simulink model "LQR_fun"  (R2018a)
settings: Solver=ode1  StartTime=0.0  StopTime=30  FixedStep=0.001  RelTol=1e-3
InitFcn:
  | lqr_main
values from neighbouring files (symbols this model uses):
  den = [1 PlantX.B/PlantX.J PlantX.K/PlantX.J]    [lqr_m.m]    (also in lqr_main.m = [1 B/J K/J])
  num = [PlantX.K/PlantX.J]    [lqr_m.m]    (also in lqr_main.m = 15548.978804)
  tra_01 = tra_01'    [tra.m]
undefined symbols (not defined in the file or in its folder): DiscIntNeverNeededParam
libraries: simulink x3
settings Model: Creator=yuxi  LastModifiedBy=yuxi

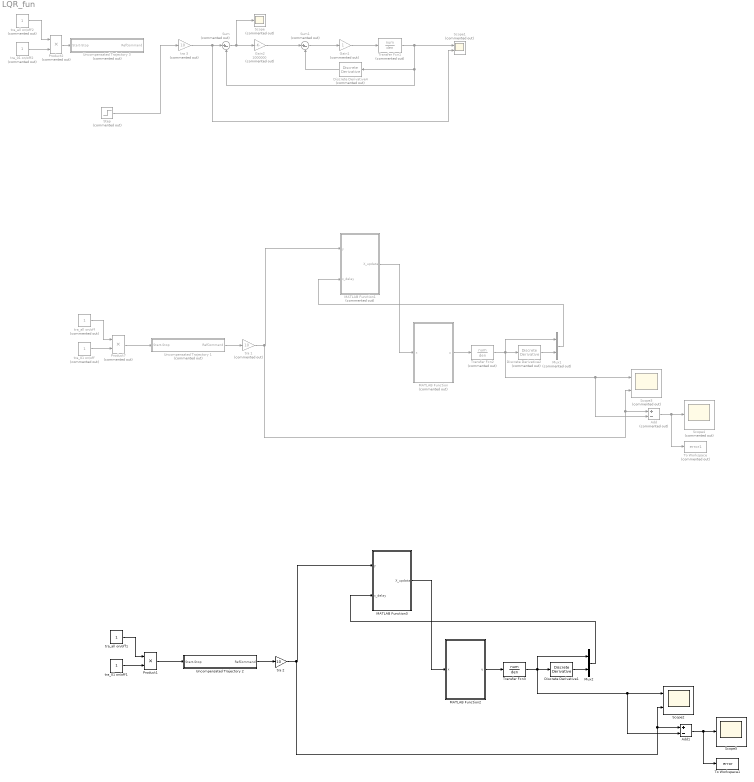
== system LQR_fun ==
  Add : Sum  Commented=on  Inputs=+-
  Add1 : Sum  Inputs=+-
  Discrete Derivative1 : simulink/Discrete/Discrete Derivative  gainval=1.0  ICPrevScaledInput=0.0  InputProcessing=Inherited  OutMin=[]  OutMax=[]  OutDataType=fixdt(1, 16)  OutScaling=2^-10  DoSatur=off
  Discrete Derivative2 : simulink/Discrete/Discrete Derivative  Commented=on  gainval=1.0  ICPrevScaledInput=0.0  InputProcessing=Inherited  OutMin=[]  OutMax=[]  OutDataType=fixdt(1, 16)  OutScaling=2^-10  DoSatur=off
  Discrete Derivative4 : simulink/Discrete/Discrete Derivative  Commented=on  gainval=1.0  ICPrevScaledInput=0.0  InputProcessing=Inherited  OutMin=[]  OutMax=[]  OutDataType=fixdt(1, 16)  OutScaling=2^-10  DoSatur=off
  Gain1 : Gain  Commented=on
  Gain2 : Gain  Commented=on  Gain=1000000
  MATLAB Function : MATLAB Function  Commented=on  TreatAsAtomicUnit=on
  MATLAB Function1 : MATLAB Function  Commented=on  TreatAsAtomicUnit=on
  MATLAB Function2 : MATLAB Function  TreatAsAtomicUnit=on
  MATLAB Function3 : MATLAB Function  TreatAsAtomicUnit=on
  Mux1 : Mux  Commented=on  Inputs=2
  Mux2 : Mux  Inputs=2
  Product1 : Product  RndMeth=Zero
  Product2 : Product  Commented=on  RndMeth=Zero
  Product7 : Product  Commented=on  RndMeth=Zero
  Scope : Scope  Commented=on
  Scope1 : Scope  Commented=on  NumInputPorts=2
  Scope2 : Scope  NumInputPorts=2
  Scope3 : Scope  Commented=on  NumInputPorts=2
  Scope4 : Scope  Commented=on
  Scope5 : Scope
  Step : Step  Commented=on  SampleTime=0
  Sum : Sum  Commented=on  Inputs=|+-
  Sum1 : Sum  Commented=on  Inputs=|+-
  To Workspace : ToWorkspace  Commented=on  VariableName=error1  SaveFormat=Timeseries  SampleTime=-1
  To Workspace1 : ToWorkspace  VariableName=error  SaveFormat=Timeseries  SampleTime=-1
  Transfer Fcn1 : TransferFcn  Commented=on  Numerator=num  Denominator=den
  Transfer Fcn2 : TransferFcn  Commented=on  Numerator=num  Denominator=den
  Transfer Fcn3 : TransferFcn  Numerator=num  Denominator=den
  Uncompensated Trajectory 1 : Subsystem  Commented=on
  Uncompensated Trajectory 2 : Subsystem
  Uncompensated Trajectory 3 : Subsystem  Commented=on
  tra 1 : Gain  Commented=on  Gain=10
  tra 2 : Gain  Gain=10
  tra 3 : Gain  Commented=on  Gain=10
  tra_01 on/off : Constant  Commented=on
  tra_01 on/off1 : Constant
  tra_01 on/off2 : Constant  Commented=on
  tra_all on/off : Constant  Commented=on
  tra_all on/off1 : Constant
  tra_all on/off2 : Constant  Commented=on
  wires:
  tra 3/1 -> Scope1/2, Sum/1
  Sum/1 -> Gain2/1, Scope/1
  Transfer Fcn1/1 -> Scope1/1, Discrete Derivative4/1, Sum/2
  tra_all on/off/1 -> Product7/1
  Uncompensated Trajectory 1/1(RefCommand) -> tra 1/1
  tra_01 on/off/1 -> Product7/2
  Product7/1 -> Uncompensated Trajectory 1/1(Start-Stop)
  tra 1/1 -> Scope3/2, Add/1, MATLAB Function1/1(y)
  MATLAB Function/1(u) -> Transfer Fcn2/1
  Mux1/1 -> MATLAB Function1/2(x_delay)
  Transfer Fcn2/1 -> Mux1/1, Discrete Derivative2/1, Add/2, Scope3/1
  MATLAB Function1/1(X_updata) -> MATLAB Function/1(x)
  Discrete Derivative2/1 -> Mux1/2
  Add/1 -> To Workspace/1, Scope4/1
  Product2/1 -> Uncompensated Trajectory 3/1(Start-Stop)
  tra_all on/off2/1 -> Product2/1
  tra_01 on/off2/1 -> Product2/2
  Step/1 -> tra 3/1
  Gain2/1 -> Sum1/1
  Discrete Derivative4/1 -> Sum1/2
  Sum1/1 -> Gain1/1
  Gain1/1 -> Transfer Fcn1/1
  tra 2/1 -> Scope2/2, Add1/1, MATLAB Function3/1(y)
  MATLAB Function3/1(X_updata) -> MATLAB Function2/1(x)
  Add1/1 -> To Workspace1/1, Scope5/1
  Uncompensated Trajectory 2/1(RefCommand) -> tra 2/1
  Discrete Derivative1/1 -> Mux2/2
  MATLAB Function2/1(u) -> Transfer Fcn3/1
  Transfer Fcn3/1 -> Mux2/1, Discrete Derivative1/1, Add1/2, Scope2/1
  tra_01 on/off1/1 -> Product1/2
  Mux2/1 -> MATLAB Function3/2(x_delay)
  Product1/1 -> Uncompensated Trajectory 2/1(Start-Stop)
  tra_all on/off1/1 -> Product1/1

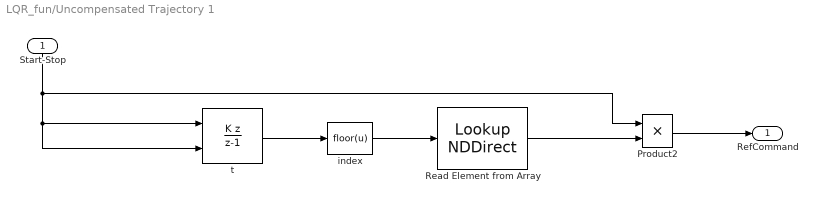
== system LQR_fun/Uncompensated Trajectory 1 ==
  Start-Stop : Inport
  Product2 : Product  RndMeth=Zero
  Read Element from Array : LookupNDDirect  NumberOfTableDimensions=1  Table=tra_01
  index : Fcn  Expr=floor(u)
  t : DiscreteIntegrator  IntegratorMethod=Accumulation: Backward Euler  ExternalReset=rising  SampleTime=-1  ICPrevOutput=DiscIntNeverNeededParam  ICPrevScaledInput=DiscIntNeverNeededParam
  RefCommand : Outport
  wires:
  Read Element from Array/1 -> Product2/2
  t/1 -> index/1
  Product2/1 -> RefCommand/1
  Start-Stop/1 -> Product2/1, t/1, t/2
  index/1 -> Read Element from Array/1

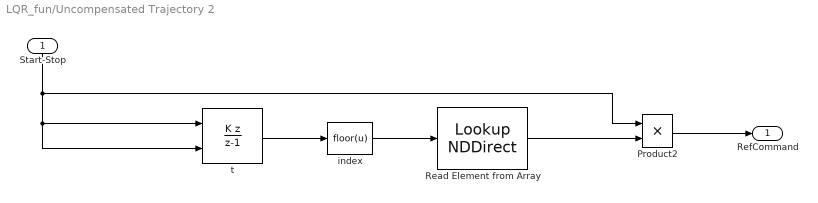
== system LQR_fun/Uncompensated Trajectory 2 ==
  Start-Stop : Inport
  Product2 : Product  RndMeth=Zero
  Read Element from Array : LookupNDDirect  NumberOfTableDimensions=1  Table=tra_01
  index : Fcn  Expr=floor(u)
  t : DiscreteIntegrator  IntegratorMethod=Accumulation: Backward Euler  ExternalReset=rising  SampleTime=-1  ICPrevOutput=DiscIntNeverNeededParam  ICPrevScaledInput=DiscIntNeverNeededParam
  RefCommand : Outport
  wires:
  Read Element from Array/1 -> Product2/2
  t/1 -> index/1
  Product2/1 -> RefCommand/1
  Start-Stop/1 -> Product2/1, t/1, t/2
  index/1 -> Read Element from Array/1

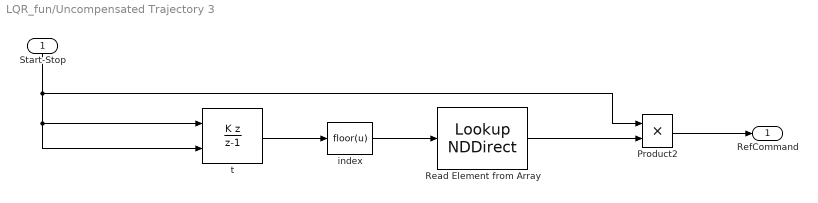
== system LQR_fun/Uncompensated Trajectory 3 ==
  Start-Stop : Inport
  Product2 : Product  RndMeth=Zero
  Read Element from Array : LookupNDDirect  NumberOfTableDimensions=1  Table=tra_01
  index : Fcn  Expr=floor(u)
  t : DiscreteIntegrator  IntegratorMethod=Accumulation: Backward Euler  ExternalReset=rising  SampleTime=-1  ICPrevOutput=DiscIntNeverNeededParam  ICPrevScaledInput=DiscIntNeverNeededParam
  RefCommand : Outport
  wires:
  Read Element from Array/1 -> Product2/2
  t/1 -> index/1
  Product2/1 -> RefCommand/1
  Start-Stop/1 -> Product2/1, t/1, t/2
  index/1 -> Read Element from Array/1

== matlab function LQR_fun/MATLAB Function1 ==
  data: y input; x_delay input; X_updata output
function X_updata = Kalman_filter(y, x_delay)

A = [-2.173321024694207,-1.214763969059581e+02;128,0];
B = [8;0];
% C = [0,15.184549613244759];
C = [1,0];

D = 0;

P = [1 0; 0 1];
Q = [0.05 0; 0 0.05];
R = 1;

x_next = A*x_delay;
P_next = A*P*A' + Q;
K = P_next*C' / (C*P_next*C' + R);    % 卡尔曼增益(Kalman Gain)
X_updata = x_next + K*(y - C*x_next)
P_updata = (eye(2) - K*C) * P_next; 

end

== matlab function LQR_fun/MATLAB Function ==
  data: x input; u output
function u  = LQR(x)
% function u  = LQR(x)

% PlantX.J = 0.00004333;     %(kg*m^2)
% PlantX.B = 0.00009417;      %(kg*m^2/s)
% PlantX.Ka = 0.8268;       %(A/V)
% PlantX.Kt = 0.512;       %Nm/A
% PlantX.rg = 10/(2*pi);         %mm/rad
% PlantX.K = PlantX.Ka*PlantX.Kt*PlantX.rg;   %(N*m^2/V)/1000
% num = [PlantX.K/PlantX.J];
% den = [1 PlantX.B/PlantX.J PlantX.K/PlantX.J];

% sys = tf(num, den);
% [A B C D] = ssdata(sys);

coder.extrinsic('lqr');

A = [-2.173321024694207,-1.214763969059581e+02;128,0];
B = [8;0];
C = [0,15.184549613244759];
D = 0;
 
Q = [0.18 0; 0 0.15];
R = 1;
% Q = [0.01 0; 0 0.01];
% R = 1;

K = zeros(1,2);
K = lqr(A,B,Q,R);
u = K*x;    % x(2X1);u(1X1)

% u_temp = K*x;
% u = [u_temp;0];

end

== matlab function LQR_fun/MATLAB Function2 ==
  data: x input; u output
function u  = LQR(x)
% function u  = LQR(x)

% PlantX.J = 0.00004333;     %(kg*m^2)
% PlantX.B = 0.00009417;      %(kg*m^2/s)
% PlantX.Ka = 0.8268;       %(A/V)
% PlantX.Kt = 0.512;       %Nm/A
% PlantX.rg = 10/(2*pi);         %mm/rad
% PlantX.K = PlantX.Ka*PlantX.Kt*PlantX.rg;   %(N*m^2/V)/1000
% num = [PlantX.K/PlantX.J];
% den = [1 PlantX.B/PlantX.J PlantX.K/PlantX.J];

% sys = tf(num, den);
% [A B C D] = ssdata(sys);

coder.extrinsic('lqr');

A = [-2.173321024694207,-1.214763969059581e+02;128,0];
B = [8;0];
C = [0,15.184549613244759];
D = 0;
 
Q = [0.18 0; 0 0.15];
R = 1;

K = zeros(1,2);
K = lqr(A,B,Q,R);
u = K*x;    % x(2X1);u(1X1)

% u_temp = K*x;
% u = [u_temp;0];

end

== matlab function LQR_fun/MATLAB Function3 ==
  data: y input; x_delay input; X_updata output
function X_updata = Kalman_filter(y, x_delay)

% y =1;
% x_delay = [0.9, 1]';

A = [-2.173321024694207,-1.214763969059581e+02;128,0];
B = [8;0];
% C = [0,15.184549613244759];
C = [1 0];
D = 0;

P = [1 0; 0 1];
Q = [0.05 0; 0 0.05];
R = 1;

x_next = A*x_delay;
P_next = A*P*A' + Q;
K = P_next*C' / (C*P_next*C' + R);    % 卡尔曼增益(Kalman Gain)
X_updata = x_next + K*(y - C*x_next)
P_updata = (eye(2) - K*C) * P_next; 

end
